simulink model "pi_seudoControllerBallandBeam"  (R2024a)
settings: Solver=VariableStepAuto  StartTime=0.0  StopTime=10.0  RelTol=1e-3
undefined symbols (not defined in the file or in its folder): a, GP_den, GP_num, KD, KI, KP
settings Model: Creator=ASHISH KUMAR SINGH  LastModifiedBy=ASHISH KUMAR SINGH

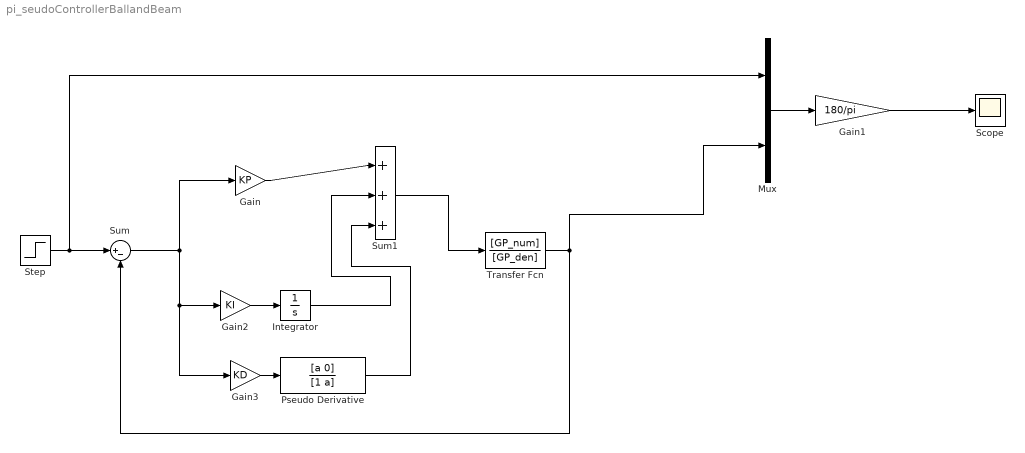
== system pi_seudoControllerBallandBeam ==
  Gain : Gain  Gain=KP
  Gain1 : Gain  Gain=180/pi
  Gain2 : Gain  Gain=KI
  Gain3 : Gain  Gain=KD
  Integrator : Integrator
  Mux : Mux  Inputs=2
  Pseudo Derivative : TransferFcn  Numerator=[a 0]  Denominator=[1 a]
  Scope : Scope
  Step : Step  SampleTime=0
  Sum : Sum  Inputs=|+-
  Sum1 : Sum  Inputs=|+++
  Transfer Fcn : TransferFcn  Numerator=[GP_num]  Denominator=[GP_den]
  wires:
  Transfer Fcn/1 -> Sum/2, Mux/2
  Gain1/1 -> Scope/1
  Pseudo Derivative/1 -> Sum1/3
  Sum/1 -> Gain/1, Gain3/1, Gain2/1
  Gain3/1 -> Pseudo Derivative/1
  Mux/1 -> Gain1/1
  Gain/1 -> Sum1/1
  Gain2/1 -> Integrator/1
  Sum1/1 -> Transfer Fcn/1
  Integrator/1 -> Sum1/2
  Step/1 -> Mux/1, Sum/1
